simulink model "BLDCmotorControl_FOC_R2017b_fixdt_Ffwd"  (R2017b)
settings: Solver=FixedStepDiscrete  StartTime=0  StopTime=0.5  FixedStep=Ts  MaxStep=1e-6  RelTol=1e-6  AbsTol=1e-6  EnableMultiTasking=on
PreLoadFcn:
  | addpath(genpath('01_Libraries'));
  | addpath(genpath('02_Figures'));
InitFcn:
  | init_model;
values from neighbouring files (symbols this model uses):
  a_elecAngle = 60    [init_model_Ffwd.m]
  b_DCLinkCurrAvail = 0    [init_model_Ffwd.m]
  b_diagEna = 1    [init_model_Ffwd.m]
  b_FfwdEna = 1    [init_model_Ffwd.m]
  b_fieldWeakEna = 0    [init_model_Ffwd.m]
  b_selPhaABCurrMeas = 1    [init_model_Ffwd.m]
  cf_currFilt = 0.02    [init_model_Ffwd.m]
  cf_speedCoef = round(f_ctrl * a_mechAngle * (pi/180) * (30/pi))    [init_model_Ffwd.m]
  cf_speedFilt = 0.20    (= 0.2)    [init_model_Ffwd.m]
  CTRL_COM = 0    [init_model_Ffwd.m]
  dV_openRate = 1000 * Ts_ctrl    (= 0.06)    [init_model_Ffwd.m]
  dz_cntTrnsDetHi = 40    [init_model_Ffwd.m]
  dz_cntTrnsDetLo = 20    [init_model_Ffwd.m]
  i_errThres = 40 * i_sca    (= 2000)    [init_model_Ffwd.m]
  i_max = i_max * i_sca    (= 750)    [init_model_Ffwd.m]
  i_thresOutlier = 200    [init_model_Ffwd.m]
  id_fieldWeak_M1 = [  0   0  0.05  0.25    1    2    3    4  4.5  4.8   5   5] * i_sca    [init_model_Ffwd.m]
  id_Kb = 1000 * Ts_ctrl    (= 0.06)    [init_model_Ffwd.m]
  id_Ki = 80 * Ts_ctrl    (= 0.0048)    [init_model_Ffwd.m]
  id_Kp = 0.5    [init_model_Ffwd.m]
  iq_Kb = 1000 * Ts_ctrl    (= 0.06)    [init_model_Ffwd.m]
  iq_Ki = 100 * Ts_ctrl    (= 0.006)    [init_model_Ffwd.m]
  iq_KiLimProt = 3 * Ts_ctrl    (= 0.00018)    [init_model_Ffwd.m]
  iq_Kp = 0.5    [init_model_Ffwd.m]
  iq_KpLimProt = 4    [init_model_Ffwd.m]
  iq_max_M1 = sqrt(i_max^2 - iq_max_XA.^2)    [init_model_Ffwd.m]
  Ld = 0.00024368    [pe_electric_engine_dyno_data.m]
  Lq = 0.00029758    [pe_electric_engine_dyno_data.m]
  mot_lambda = 0    [init_model_Ffwd.m]
  mot_Ld = 0    [init_model_Ffwd.m]
  mot_Lq = 0    [init_model_Ffwd.m]
  n_commAcvLo = 15    [init_model_Ffwd.m]
  n_commDeacvHi = 30    [init_model_Ffwd.m]
  n_Kb = 1000 * Ts_ctrl    (= 0.06)    [init_model_Ffwd.m]
  n_Ki = 10 * Ts_ctrl    (= 0.0006)    [init_model_Ffwd.m]
  n_Kp = 1    [init_model_Ffwd.m]
  n_KpLimProt = 5    [init_model_Ffwd.m]
  n_max = 800    [init_model_Ffwd.m]
  n_stdStillDet = 3    [init_model_Ffwd.m]
  OPEN_MODE = 0    [init_model_Ffwd.m]
  r_cos_M1 = cos((a_elecAngle_XA + 30)*(pi/180))    [init_model_Ffwd.m]
  r_sin_M1 = sin((a_elecAngle_XA + 30)*(pi/180))    [init_model_Ffwd.m]
  r_whl = 6.5 * 2.54 * 1e-2 / 2    (= 0.08255)    [init_model_Ffwd.m]
  Rs = 0.010087    [pe_electric_engine_dyno_data.m]
  SPD_MODE = 2    [init_model_Ffwd.m]
  t_errDequal = 2 * f_ctrl    (= 32000)    [init_model_Ffwd.m]
  t_errQual = 0.8 * f_ctrl    (= 12800)    [init_model_Ffwd.m]
  TRQ_MODE = 3    [init_model_Ffwd.m]
  Ts = 5e-6    (= 5e-06)    [init_model_Ffwd.m]    (also in pe_electric_engine_dyno_data.m = 1e-05)
  Ts_ctrl = 6e-5    (= 6e-05)    [init_model_Ffwd.m]
  Vd_max = 1000 - V_margin    (= 900)    [init_model_Ffwd.m]
  vec_hallToPos = [0 2 0 1 4 3 5 0]    [init_model_Ffwd.m]
  VLT_MODE = 1    [init_model_Ffwd.m]
  Vq_max_M1 = sqrt(Vd_max^2 - Vq_max_XA.^2)    [init_model_Ffwd.m]
  z_commutMap_M1 = [-1 -1  0  1  1  0 ... (first row only)    [init_model_Ffwd.m]
  z_ctrlModReq = 1    [init_model_Ffwd.m]
  z_ctrlTypSel = 1    [init_model_Ffwd.m]
  z_maxCntRst = 2000    [init_model_Ffwd.m]
undefined symbols (not defined in the file or in its folder): DiscIntNeverNeededParam, sigbuilder_block, V_max, V_min
libraries: powerlib x14, BLDC_controller_Lib x12, simulink x11, pePwmGenerator x1
(part 3 of 3)

== system BLDCmotorControl_FOC_R2017b_fixdt_Ffwd/BLDC_controller/BLDC_controller/F04_Field_Oriented_Control/FeefForward_Decoupling ==
  note: FOC Feedforward Decoupling
      | Vq_Ffwd = n_mot * (mot_Ld*id_Tgt + mot_lambda)
      | Vd_Ffwd = -n_mot * mot_Lq * iq
  n_mot : Inport
  iq_Tgt : Inport  Port=2
  id_Tgt : Inport  Port=3
  Action Port : ActionPort  InitializeStates=reset  ActionType=then
  Divide1 : Product  Inputs=**  RndMeth=Simplest  SaturateOnIntegerOverflow=on  OutDataTypeStr=Inherit: Same as first input
  Divide2 : Product  Inputs=**  OutDataTypeStr=fixdt(1,16,8)  RndMeth=Simplest
  Divide3 : Product  Inputs=**  RndMeth=Simplest  SaturateOnIntegerOverflow=on  OutDataTypeStr=Inherit: Same as first input
  Divide4 : Product  Inputs=**  OutDataTypeStr=fixdt(1,16,8)  RndMeth=Simplest
  Sum6 : Sum  OutDataTypeStr=fixdt(1,16,7)  RndMeth=Simplest
  mot_Ld : Constant  Value=mot_Ld  OutDataTypeStr=fixdt(0,16,16)
  mot_Lq : Constant  Value=mot_Lq  OutDataTypeStr=fixdt(0,16,16)
  mot_lambda : Constant  Value=mot_lambda  OutDataTypeStr=fixdt(0,16,9)
  toNegative : Gain  Tag=struct('comment',struct('text','','placement',1),'logdata',struct('maxnumvals',inf,'plotchannels',[],'loggingmode',3,'channels',1),'output',struct('variable','','description','','name','$S_$B','width',1,'address','','max',NaN,'min',NaN,'class','default','type','CONTINUOUS','scaling','','lsb',1,'offset',0,'arb',0,'freeze',1,'unit','','autoscalingmode',1,'lowerheadroom',1,'upperheadroom',1,'headroomunit','bit','keepdatatype',1,'checkmin',0,'checkmax',0,'castoutput',0,'show',0),'gain',struct('variable','','description','','name','$S_$B_gain','width',1,'address','','max',NaN,'min',NaN,'class','default','type','CONTINUOUS','scaling','','lsb',1,'offset',0,'arb',0,'freeze',1,'unit','','keepdatatype',1,'value','1','scalar',0,'tolerance',1),'scalingvalid',0,'date',730486)  Gain=-1  RndMeth=Zero  OutDataTypeStr=Inherit: Same as input  ParamDataTypeStr=Inherit: Same as input
  Vq_Ffwd : Outport  OutputWhenDisabled=reset  InitialOutput=0
  Vd_Ffwd : Outport  Port=2  OutputWhenDisabled=reset  InitialOutput=0
  wires:
  n_mot/1 -> [n_mot]
  iq_Tgt/1 -> [iq_Tgt]
  id_Tgt/1 -> [id_Tgt]
  Divide1/1 -> toNegative/1
  mot_Ld/1 -> Divide2/2
  [id_Tgt] -> Divide2/1
  Divide2/1 -> Sum6/1
  toNegative/1 -> Vd_Ffwd/1
  mot_lambda/1 -> Sum6/2
  Sum6/1 -> Divide3/2
  [n_mot] -> Divide3/1
  Divide3/1 -> Vq_Ffwd/1
  mot_Lq/1 -> Divide4/2
  [n_mot] -> Divide1/1
  Divide4/1 -> Divide1/2
  [iq_Tgt] -> Divide4/1

== system BLDCmotorControl_FOC_R2017b_fixdt_Ffwd/BLDC_controller/BLDC_controller/F04_Field_Oriented_Control/Field_Weakening ==
  note: Sine/Cosine Look-up Tables
  note: FOC Field weakening
  note: Note: The Sine and Cosine maps are shifted in phase by 30 deg to align with the Hall sensors position.
  note: Field Weakening map as a function of Motor Speed
  a_elecAngle : Inport
  n_motAbs : Inport  Port=2
  Data Type Conversion : DataTypeConversion  OutDataTypeStr=fixdt(1,16,4)
  Switch1 : Switch  Criteria=u2 ~= 0  OutDataTypeStr=Inherit: Inherit via back propagation  RndMeth=Zero
  a_elecAngle_XA : PreLookup  BreakpointsData=a_elecAngle_XA  OutputSelection=Index only  IndexSearchMethod=Evenly spaced points  BeginIndexSearchUsingPreviousIndexResult=on  IndexDataTypeStr=uint8  FractionDataTypeStr=fixdt(0,16,14)  RndMeth=Simplest
  a_elecPeriod1 : Constant  Value=0  OutDataTypeStr=Inherit: Inherit via back propagation
  a_elecPeriod3 : Constant  Value=0  OutDataTypeStr=uint8
  b_fieldWeakEna : Constant  Value=b_fieldWeakEna  OutDataTypeStr=boolean
  id_fieldWeak_M1 : Interpolation_n-D  NumberOfTableDimensions=1  Table=id_fieldWeak_M1  ExtrapMethod=Clip  OutDataTypeStr=fixdt(0,10,0)  InternalRulePriority=Speed  RndMeth=Simplest
      settings: InputPortMap=u0,u1
  n_fieldWeak_XA : PreLookup  BreakpointsData=n_fieldWeak_XA  IndexSearchMethod=Evenly spaced points  BeginIndexSearchUsingPreviousIndexResult=on  IndexDataTypeStr=uint8  FractionDataTypeStr=fixdt(0,8,6)  RndMeth=Simplest
  r_cos_M1 : Interpolation_n-D  NumberOfTableDimensions=1  Table=r_cos_M1  InterpMethod=Flat  ExtrapMethod=Clip  ValidIndexMayReachLast=on  OutDataTypeStr=fixdt(1,16,14)  InternalRulePriority=Speed  RndMeth=Simplest
      settings: InputPortMap=u0,u1
  r_sin_M1 : Interpolation_n-D  NumberOfTableDimensions=1  Table=r_sin_M1  InterpMethod=Flat  ExtrapMethod=Clip  ValidIndexMayReachLast=on  OutDataTypeStr=fixdt(1,16,14)  InternalRulePriority=Speed  RndMeth=Simplest
      settings: InputPortMap=u0,u1
  toNegative : Gain  Tag=struct('comment',struct('text','','placement',1),'logdata',struct('maxnumvals',inf,'plotchannels',[],'loggingmode',3,'channels',1),'output',struct('variable','','description','','name','$S_$B','width',1,'address','','max',NaN,'min',NaN,'class','default','type','CONTINUOUS','scaling','','lsb',1,'offset',0,'arb',0,'freeze',1,'unit','','autoscalingmode',1,'lowerheadroom',1,'upperheadroom',1,'headroomunit','bit','keepdatatype',1,'checkmin',0,'checkmax',0,'castoutput',0,'show',0),'gain',struct('variable','','description','','name','$S_$B_gain','width',1,'address','','max',NaN,'min',NaN,'class','default','type','CONTINUOUS','scaling','','lsb',1,'offset',0,'arb',0,'freeze',1,'unit','','keepdatatype',1,'value','1','scalar',0,'tolerance',1),'scalingvalid',0,'date',730486)  Gain=-1  OutDataTypeStr=fixdt(1,16,4)  RndMeth=Zero  ParamDataTypeStr=Inherit: Same as input
  r_sin : Outport
  r_cos : Outport  Port=2
  id_Tgt : Outport  Port=3
  id_TgtAbs : Outport  Port=4
  wires:
  a_elecAngle_XA/1 -> r_cos_M1/1, r_sin_M1/1
  r_sin_M1/1 -> r_sin/1
  a_elecAngle/1 -> a_elecAngle_XA/1
  r_cos_M1/1 -> r_cos/1
  a_elecPeriod3/1 -> r_cos_M1/2, r_sin_M1/2
  n_fieldWeak_XA/1 -> id_fieldWeak_M1/1
  id_fieldWeak_M1/1 -> Data Type Conversion/1
  n_fieldWeak_XA/2 -> id_fieldWeak_M1/2
  b_fieldWeakEna/1 -> Switch1/2
  Switch1/1 -> id_TgtAbs/1, toNegative/1
  Data Type Conversion/1 -> Switch1/1
  a_elecPeriod1/1 -> Switch1/3
  n_motAbs/1 -> n_fieldWeak_XA/1
  toNegative/1 -> id_Tgt/1

== system BLDCmotorControl_FOC_R2017b_fixdt_Ffwd/BLDC_controller/BLDC_controller/F04_Field_Oriented_Control/Inv_Clarke_Transform ==
  note: Inverse Clarke Transform:
      | V_phaA = V_alpha
      | V_phaB = -(1/2)*V_alpha + (sqrt(3)/2)*V_beta
      | V_phaC = -VphaA - V_phaB
  note: Space Vector Modulation (SVM)
  V_alpha : Inport
  V_beta : Inport  Port=2
  Add : Sum
  Add1 : Sum  Inputs=-+  OutDataTypeStr=Inherit: Same as first input
  Demux : Demux  Outputs=3
  Gain1 : Gain  Tag=struct('comment',struct('text','','placement',1),'logdata',struct('maxnumvals',inf,'plotchannels',[],'loggingmode',3,'channels',1),'output',struct('variable','','description','','name','$S_$B','width',1,'address','','max',NaN,'min',NaN,'class','default','type','CONTINUOUS','scaling','','lsb',1,'offset',0,'arb',0,'freeze',1,'unit','','autoscalingmode',1,'lowerheadroom',1,'upperheadroom',1,'headroomunit','bit','keepdatatype',1,'checkmin',0,'checkmax',0,'castoutput',0,'show',0),'gain',struct('variable','','description','','name','$S_$B_gain','width',1,'address','','max',NaN,'min',NaN,'class','default','type','CONTINUOUS','scaling','','lsb',1,'offset',0,'arb',0,'freeze',1,'unit','','keepdatatype',1,'value','1','scalar',0,'tolerance',1),'scalingvalid',0,'date',730486)  Gain=sqrt(3)/2  OutDataTypeStr=fixdt(1,16,5)  RndMeth=Zero
  Gain2 : Gain  Gain=0.5  OutDataTypeStr=Inherit: Same as input
  Gain3 : Gain  Tag=struct('comment',struct('text','','placement',1),'logdata',struct('maxnumvals',inf,'plotchannels',[],'loggingmode',3,'channels',1),'output',struct('variable','','description','','name','$S_$B','width',1,'address','','max',NaN,'min',NaN,'class','default','type','CONTINUOUS','scaling','','lsb',1,'offset',0,'arb',0,'freeze',1,'unit','','autoscalingmode',1,'lowerheadroom',1,'upperheadroom',1,'headroomunit','bit','keepdatatype',1,'checkmin',0,'checkmax',0,'castoutput',0,'show',0),'gain',struct('variable','','description','','name','$S_$B_gain','width',1,'address','','max',NaN,'min',NaN,'class','default','type','CONTINUOUS','scaling','','lsb',1,'offset',0,'arb',0,'freeze',1,'unit','','keepdatatype',1,'value','1','scalar',0,'tolerance',1),'scalingvalid',0,'date',730486)  Gain=1/2  OutDataTypeStr=fixdt(1,16,5)  RndMeth=Zero
  Gain4 : Gain  Gain=2/sqrt(3)  OutDataTypeStr=fixdt(1,16,0)
  MinMax1 : MinMax  InputSameDT=on
  MinMax2 : MinMax  Function=max  InputSameDT=on
  Mux4 : Mux  Inputs=3
  Sum2 : Sum  Inputs=--  OutDataTypeStr=fixdt(1,16,4)  RndMeth=Simplest
  Sum6 : Sum  Inputs=-+  OutDataTypeStr=fixdt(1,16,4)  RndMeth=Simplest
  V_phaA : Outport
  V_phaB : Outport  Port=2
  V_phaC : Outport  Port=3
  wires:
  Sum6/1 -> Sum2/2, Mux4/2
  Sum2/1 -> Mux4/3
  Gain1/1 -> Sum6/2
  Gain3/1 -> Sum6/1
  V_alpha/1 -> Gain3/1, Sum2/1, Mux4/1  "alpha"
  V_beta/1 -> Gain1/1  "beta"
  Add/1 -> Gain2/1
  Add1/1 -> Gain4/1
  MinMax1/1 -> Add/1
  Demux/3 -> V_phaC/1
  Demux/2 -> V_phaB/1
  Gain2/1 -> Add1/1
  Demux/1 -> V_phaA/1
  MinMax2/1 -> Add/2
  Mux4/1 -> Add1/2, MinMax2/1, MinMax1/1
  Gain4/1 -> Demux/1

== system BLDCmotorControl_FOC_R2017b_fixdt_Ffwd/BLDC_controller/BLDC_controller/F04_Field_Oriented_Control/Inv_Park_Transform ==
  note: Inverse Park Transform:
      | V_alpha = Vd*cos(angle) - Vq*sin(angle)
      | V_beta = Vd*sin(angle) + Vq*cos(angle)
  Vq : Inport
  Vd : Inport  Port=2
  r_sin : Inport  Port=3
  r_cos : Inport  Port=4
  Divide{1..4} (4 alike) : Product  Inputs=**  OutDataTypeStr=fixdt(1,16,5)  RndMeth=Simplest
  Sum1 : Sum  OutDataTypeStr=fixdt(1,16,4)  RndMeth=Simplest
  Sum6 : Sum  Inputs=+-  OutDataTypeStr=fixdt(1,16,4)  RndMeth=Simplest
  V_alpha : Outport
  V_beta : Outport  Port=2
  wires:
  r_sin/1 -> [r_sin]
  Vd/1 -> [Vd]
  Vq/1 -> [Vq]
  r_cos/1 -> [r_cos]
  [r_cos] -> Divide4/2
  [r_sin] -> Divide1/2
  [Vd] -> Divide4/1
  [r_cos] -> Divide3/2
  Divide1/1 -> Sum6/2
  [Vq] -> Divide1/1
  [Vd] -> Divide2/1
  Divide2/1 -> Sum1/1
  Divide3/1 -> Sum1/2
  [Vq] -> Divide3/1
  Divide4/1 -> Sum6/1
  [r_sin] -> Divide2/2
  Sum1/1 -> V_beta/1
  Sum6/1 -> V_alpha/1

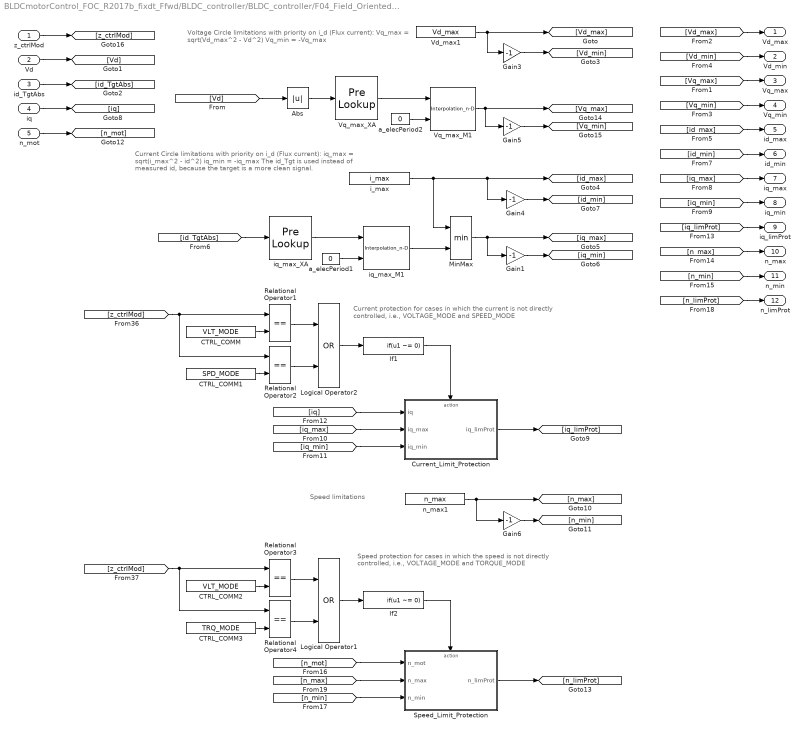
== system BLDCmotorControl_FOC_R2017b_fixdt_Ffwd/BLDC_controller/BLDC_controller/F04_Field_Oriented_Control/Motor_Limitations ==
  note: Voltage Circle limitations with priority on i_d (Flux current):
      | Vq_max = sqrt(Vd_max^2 - Vd^2)
      | Vq_min = -Vq_max
  note: Current Circle limitations with priority on i_d (Flux current):
      | iq_max = sqrt(i_max^2 - id^2)
      | iq_min = -iq_max
      |
      | The id_Tgt is used instead of measured id, because the target is a more clean signal.
  note: Speed limitations
  note: Current protection
      | for cases in which the current is not directly controlled, i.e., VOLTAGE_MODE and SPEED_MODE
  note: Speed protection
      | for cases in which the speed is not directly controlled, i.e., VOLTAGE_MODE and TORQUE_MODE
  z_ctrlMod : Inport
  Vd : Inport  Port=2
  id_TgtAbs : Inport  Port=3
  iq : Inport  Port=4
  n_mot : Inport  Port=5
  Abs : Abs
  CTRL_COMM : Constant  Value=VLT_MODE  OutDataTypeStr=Inherit: Inherit via back propagation
  CTRL_COMM1 : Constant  Value=SPD_MODE  OutDataTypeStr=Inherit: Inherit via back propagation
  CTRL_COMM2 : Constant  Value=VLT_MODE  OutDataTypeStr=Inherit: Inherit via back propagation
  CTRL_COMM3 : Constant  Value=TRQ_MODE  OutDataTypeStr=Inherit: Inherit via back propagation
  Current_Limit_Protection : Subsystem
  Gain{1,3..6} (5 alike) : Gain  Tag=struct('comment',struct('text','','placement',1),'logdata',struct('maxnumvals',inf,'plotchannels',[],'loggingmode',3,'channels',1),'output',struct('variable','','description','','name','$S_$B','width',1,'address','','max',NaN,'min',NaN,'class','default','type','CONTINUOUS','scaling','','lsb',1,'offset',0,'arb',0,'freeze',1,'unit','','autoscalingmode',1,'lowerheadroom',1,'upperheadroom',1,'headroomunit','bit','keepdatatype',1,'checkmin',0,'checkmax',0,'castoutput',0,'show',0),'gain',struct('variable','','description','','name','$S_$B_gain','width',1,'address','','max',NaN,'min',NaN,'class','default','type','CONTINUOUS','scaling','','lsb',1,'offset',0,'arb',0,'freeze',1,'unit','','keepdatatype',1,'value','1','scalar',0,'tolerance',1),'scalingvalid',0,'date',730486)  Gain=-1  RndMeth=Zero  OutDataTypeStr=Inherit: Same as input  ParamDataTypeStr=Inherit: Same as input
  If1 : If  IfExpression=u1 ~= 0  ShowElse=off
  If2 : If  IfExpression=u1 ~= 0  ShowElse=off
  Logical Operator1 : Logic  Operator=OR  AllPortsSameDT=off  OutDataTypeStr=boolean
  Logical Operator2 : Logic  Operator=OR  AllPortsSameDT=off  OutDataTypeStr=boolean
  MinMax : MinMax  Inputs=2
  Relational Operator{1..4} (4 alike) : RelationalOperator  Operator===  OutDataTypeStr=boolean  RndMeth=Simplest
  Speed_Limit_Protection : Subsystem
  Vd_max1 : Constant  Value=Vd_max  OutDataTypeStr=fixdt(1,16,4)
  Vq_max_M1 : Interpolation_n-D  NumberOfTableDimensions=1  Table=Vq_max_M1  InterpMethod=Flat  ExtrapMethod=Clip  ValidIndexMayReachLast=on  OutDataTypeStr=fixdt(1,16,4)  InternalRulePriority=Speed  RndMeth=Simplest
      settings: InputPortMap=u0,u1
  Vq_max_XA : PreLookup  BreakpointsData=Vq_max_XA  OutputSelection=Index only  IndexSearchMethod=Evenly spaced points  BeginIndexSearchUsingPreviousIndexResult=on  IndexDataTypeStr=uint8  FractionDataTypeStr=fixdt(0,8,6)  RndMeth=Simplest
  a_elecPeriod1 : Constant  Value=0  OutDataTypeStr=uint8
  a_elecPeriod2 : Constant  Value=0  OutDataTypeStr=uint8
  i_max : Constant  Value=i_max  OutDataTypeStr=fixdt(1,16,4)
  iq_max_M1 : Interpolation_n-D  NumberOfTableDimensions=1  Table=iq_max_M1  InterpMethod=Flat  ExtrapMethod=Clip  ValidIndexMayReachLast=on  OutDataTypeStr=fixdt(1,16,4)  InternalRulePriority=Speed  RndMeth=Simplest
      settings: InputPortMap=u0,u1
  iq_max_XA : PreLookup  BreakpointsData=iq_max_XA  OutputSelection=Index only  IndexSearchMethod=Evenly spaced points  BeginIndexSearchUsingPreviousIndexResult=on  IndexDataTypeStr=uint8  FractionDataTypeStr=fixdt(0,8,6)  RndMeth=Simplest
  n_max1 : Constant  Value=n_max  OutDataTypeStr=fixdt(1,16,4)
  Vd_max : Outport  OutputWhenDisabled=reset  InitialOutput=V_max
  Vd_min : Outport  Port=2  OutputWhenDisabled=reset  InitialOutput=V_min
  Vq_max : Outport  Port=3  OutputWhenDisabled=reset  InitialOutput=V_max
  Vq_min : Outport  Port=4  OutputWhenDisabled=reset  InitialOutput=V_min
  id_max : Outport  Port=5  OutputWhenDisabled=reset  InitialOutput=V_max
  id_min : Outport  Port=6  OutputWhenDisabled=reset  InitialOutput=V_min
  iq_max : Outport  Port=7  OutputWhenDisabled=reset  InitialOutput=V_max
  iq_min : Outport  Port=8  OutputWhenDisabled=reset  InitialOutput=V_min
  iq_limProt : Outport  Port=9  OutputWhenDisabled=reset  InitialOutput=V_min
  n_max : Outport  Port=10  OutputWhenDisabled=reset  InitialOutput=V_max
  n_min : Outport  Port=11  OutputWhenDisabled=reset  InitialOutput=V_min
  n_limProt : Outport  Port=12  OutputWhenDisabled=reset  InitialOutput=V_min
  wires:
  Vq_max_XA/1 -> Vq_max_M1/1
  [Vq_min] -> Vq_min/1
  [Vq_max] -> Vq_max/1
  Gain5/1 -> [Vq_min]
  Vd_max1/1 -> Gain3/1, [Vd_max]
  Abs/1 -> Vq_max_XA/1
  Vd/1 -> [Vd]
  [Vd] -> Abs/1
  id_TgtAbs/1 -> [id_TgtAbs]
  [Vd_max] -> Vd_max/1
  [Vd_min] -> Vd_min/1
  Gain3/1 -> [Vd_min]
  Gain4/1 -> [id_min]
  i_max/1 -> MinMax/1, Gain4/1, [id_max]
  [id_TgtAbs] -> iq_max_XA/1
  MinMax/1 -> [iq_max], Gain1/1
  Gain1/1 -> [iq_min]
  iq_max_XA/1 -> iq_max_M1/1
  [id_min] -> id_min/1
  [id_max] -> id_max/1
  [iq_max] -> iq_max/1
  [iq_min] -> iq_min/1
  iq/1 -> [iq]
  [iq_limProt] -> iq_limProt/1
  n_max1/1 -> [n_max], Gain6/1
  Gain6/1 -> [n_min]
  [n_min] -> n_min/1
  [n_max] -> n_max/1
  n_mot/1 -> [n_mot]
  [n_limProt] -> n_limProt/1
  z_ctrlMod/1 -> [z_ctrlMod]
  Relational Operator1/1 -> Logical Operator2/1
  [z_ctrlMod] -> Relational Operator2/1, Relational Operator1/1
  Logical Operator2/1 -> If1/1
  Relational Operator2/1 -> Logical Operator2/2
  CTRL_COMM/1 -> Relational Operator1/2
  CTRL_COMM1/1 -> Relational Operator2/2
  CTRL_COMM3/1 -> Relational Operator4/2
  CTRL_COMM2/1 -> Relational Operator3/2
  Relational Operator4/1 -> Logical Operator1/2
  Logical Operator1/1 -> If2/1
  [z_ctrlMod] -> Relational Operator3/1, Relational Operator4/1
  Relational Operator3/1 -> Logical Operator1/1
  [iq_max] -> Current_Limit_Protection/2(iq_max)
  [iq] -> Current_Limit_Protection/1(iq)
  [iq_min] -> Current_Limit_Protection/3(iq_min)
  Current_Limit_Protection/1(iq_limProt) -> [iq_limProt]
  [n_max] -> Speed_Limit_Protection/2(n_max)
  [n_mot] -> Speed_Limit_Protection/1(n_mot)
  [n_min] -> Speed_Limit_Protection/3(n_min)
  Speed_Limit_Protection/1(n_limProt) -> [n_limProt]
  If1/1 -> Current_Limit_Protection/Action
  If2/1 -> Speed_Limit_Protection/Action
  iq_max_M1/1 -> MinMax/2
  a_elecPeriod1/1 -> iq_max_M1/2
  Vq_max_M1/1 -> Gain5/1, [Vq_max]
  a_elecPeriod2/1 -> Vq_max_M1/2

== system BLDCmotorControl_FOC_R2017b_fixdt_Ffwd/BLDC_controller/BLDC_controller/F04_Field_Oriented_Control/Open_Mode ==
  note: This will reduce the control command to 0 with a predefined rate.
  Vq_prev : Inport
  Action Port : ActionPort  InitializeStates=reset  ActionType=default
  Constant23 : Constant  Value=0  OutDataTypeStr=Inherit: Inherit via back propagation
  Data Type Conversion : DataTypeConversion  OutDataTypeStr=fixdt(1,28,16)
  Data Type Conversion1 : DataTypeConversion  OutDataTypeStr=fixdt(1,16,4)
  Gain3 : Gain  Tag=struct('comment',struct('text','','placement',1),'logdata',struct('maxnumvals',inf,'plotchannels',[],'loggingmode',3,'channels',1),'output',struct('variable','','description','','name','$S_$B','width',1,'address','','max',NaN,'min',NaN,'class','default','type','CONTINUOUS','scaling','','lsb',1,'offset',0,'arb',0,'freeze',1,'unit','','autoscalingmode',1,'lowerheadroom',1,'upperheadroom',1,'headroomunit','bit','keepdatatype',1,'checkmin',0,'checkmax',0,'castoutput',0,'show',0),'gain',struct('variable','','description','','name','$S_$B_gain','width',1,'address','','max',NaN,'min',NaN,'class','default','type','CONTINUOUS','scaling','','lsb',1,'offset',0,'arb',0,'freeze',1,'unit','','keepdatatype',1,'value','1','scalar',0,'tolerance',1),'scalingvalid',0,'date',730486)  Gain=-1  RndMeth=Zero  OutDataTypeStr=Inherit: Same as input
  Rate_Limiter : BLDC_controller_Lib/Rate_Limiter  SystemSampleTime=-1
  dV_openRate : Constant  Value=dV_openRate  OutDataTypeStr=fixdt(1,28,16)
  rising_edge_init : BLDC_controller_Lib/rising_edge_init
  Vq_Open : Outport
  wires:
  Vq_prev/1 -> [Vq_prev]
  Constant23/1 -> Rate_Limiter/1
  rising_edge_init/1 -> Rate_Limiter/3
  Gain3/1 -> Rate_Limiter/5
  dV_openRate/1 -> Gain3/1, Rate_Limiter/4
  Data Type Conversion1/1 -> [Vq_Open]
  [Vq_Open] -> Vq_Open/1
  Rate_Limiter/1 -> Data Type Conversion1/1
  [Vq_prev] -> Data Type Conversion/1
  Data Type Conversion/1 -> Rate_Limiter/2

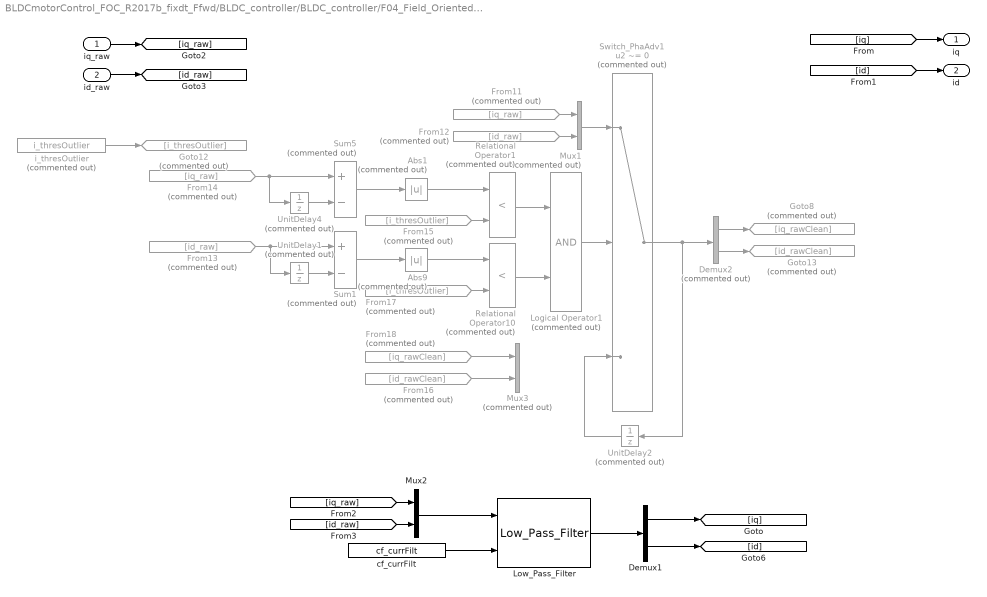
== system BLDCmotorControl_FOC_R2017b_fixdt_Ffwd/BLDC_controller/BLDC_controller/F04_Field_Oriented_Control/Outliers_Removal_and_Filtering ==
  iq_raw : Inport
  id_raw : Inport  Port=2
  Abs1 : Abs  Commented=on
  Abs9 : Abs  Commented=on
  Demux1 : Demux  Outputs=2
  Demux2 : Demux  Commented=on  Outputs=2
  From11 : From  Commented=on  GotoTag=iq_raw
  From12 : From  Commented=on  GotoTag=id_raw
  From13 : From  Commented=on  GotoTag=id_raw
  From14 : From  Commented=on  GotoTag=iq_raw
  From15 : From  Commented=on  GotoTag=i_thresOutlier
  From16 : From  Commented=on  GotoTag=id_rawClean
  From17 : From  Commented=on  GotoTag=i_thresOutlier
  From18 : From  Commented=on  GotoTag=iq_rawClean
  Goto12 : Goto  Commented=on  GotoTag=i_thresOutlier
  Goto13 : Goto  Commented=on  GotoTag=id_rawClean
  Goto8 : Goto  Commented=on  GotoTag=iq_rawClean
  Logical Operator1 : Logic  Commented=on  AllPortsSameDT=off  OutDataTypeStr=boolean
  Low_Pass_Filter : BLDC_controller_Lib/Low_Pass_Filter  SystemSampleTime=-1
  Mux1 : Mux  Commented=on  Inputs=2
  Mux2 : Mux  Inputs=2
  Mux3 : Mux  Commented=on  Inputs=2
  Relational Operator1 : RelationalOperator  Commented=on  Operator=<  OutDataTypeStr=boolean  RndMeth=Simplest
  Relational Operator10 : RelationalOperator  Commented=on  Operator=<  OutDataTypeStr=boolean  RndMeth=Simplest
  Sum1 : Sum  Commented=on  Inputs=+-  RndMeth=Simplest
  Sum5 : Sum  Commented=on  Inputs=+-  RndMeth=Simplest
  Switch_PhaAdv1 : Switch  Commented=on  Criteria=u2 ~= 0  OutDataTypeStr=Inherit: Inherit via back propagation  RndMeth=Zero
  UnitDelay1 : UnitDelay  Commented=on  SampleTime=-1
      settings: AttributesFormatString=Ini=%<X0>
  UnitDelay2 : UnitDelay  Commented=on  SampleTime=-1
      settings: AttributesFormatString=Ini=%<X0>
  UnitDelay4 : UnitDelay  Commented=on  SampleTime=-1
      settings: AttributesFormatString=Ini=%<X0>
  cf_currFilt : Constant  Value=cf_currFilt  OutDataTypeStr=fixdt(0,16,16)
  i_thresOutlier : Constant  Commented=on  Value=i_thresOutlier  OutDataTypeStr=fixdt(0,16,0)
  iq : Outport
  id : Outport  Port=2
  wires:
  Mux2/1 -> Low_Pass_Filter/1
  Sum1/1 -> Abs9/1
  Demux1/2 -> [id]
  cf_currFilt/1 -> Low_Pass_Filter/2
  UnitDelay4/1 -> Sum5/2
  UnitDelay2/1 -> Switch_PhaAdv1/3
  Abs1/1 -> Relational Operator1/1
  From17/1 -> Relational Operator10/2
  Relational Operator1/1 -> Logical Operator1/1
  Abs9/1 -> Relational Operator10/1
  Demux2/1 -> Goto8/1
  Switch_PhaAdv1/1 -> UnitDelay2/1, Demux2/1
  Demux2/2 -> Goto13/1
  From14/1 -> UnitDelay4/1, Sum5/1
  UnitDelay1/1 -> Sum1/2
  i_thresOutlier/1 -> Goto12/1
  From16/1 -> Mux3/2
  Mux1/1 -> Switch_PhaAdv1/1
  From15/1 -> Relational Operator1/2
  From12/1 -> Mux1/2
  From13/1 -> UnitDelay1/1, Sum1/1
  From11/1 -> Mux1/1
  id_raw/1 -> [id_raw]
  Relational Operator10/1 -> Logical Operator1/2
  Logical Operator1/1 -> Switch_PhaAdv1/2
  From18/1 -> Mux3/1
  [iq] -> iq/1
  [id] -> id/1
  iq_raw/1 -> [iq_raw]
  Sum5/1 -> Abs1/1
  Demux1/1 -> [iq]
  Low_Pass_Filter/1 -> Demux1/1
  [iq_raw] -> Mux2/1
  [id_raw] -> Mux2/2

== system BLDCmotorControl_FOC_R2017b_fixdt_Ffwd/BLDC_controller/BLDC_controller/F04_Field_Oriented_Control/Park_Transform ==
  note: Park Transform:
      | iq = -i_alpha*sin(angle) + i_beta*cos(angle)
      | id = i_alpha*cos(angle) + i_beta*sin(angle)
  i_apha : Inport
  i_beta : Inport  Port=2
  r_sin : Inport  Port=3
  r_cos : Inport  Port=4
  Divide{1..4} (4 alike) : Product  Inputs=**  RndMeth=Simplest  OutDataTypeStr=Inherit: Same as first input
  Sum1 : Sum  OutDataTypeStr=fixdt(1,16,4)  RndMeth=Simplest  SaturateOnIntegerOverflow=on
  Sum6 : Sum  Inputs=-+  OutDataTypeStr=fixdt(1,16,4)  RndMeth=Simplest  SaturateOnIntegerOverflow=on
  iq : Outport
  id : Outport  Port=2
  wires:
  r_sin/1 -> [r_sin]
  i_beta/1 -> [i_beta]
  i_apha/1 -> [i_apha]
  r_cos/1 -> [r_cos]
  [r_sin] -> Divide4/2
  [i_apha] -> Divide4/1
  Divide4/1 -> Sum6/1
  Divide1/1 -> Sum6/2
  [i_beta] -> Divide1/1
  [r_cos] -> Divide1/2
  Sum6/1 -> iq/1
  Divide2/1 -> Sum1/1
  [i_apha] -> Divide2/1
  [r_cos] -> Divide2/2
  Divide3/1 -> Sum1/2
  [i_beta] -> Divide3/1
  [r_sin] -> Divide3/2
  Sum1/1 -> id/1

== system BLDCmotorControl_FOC_R2017b_fixdt_Ffwd/BLDC_controller/BLDC_controller/F04_Field_Oriented_Control/Speed_Mode ==
  note: This product is necessary because the value is an input to the Integral part of the PI controller
  r_inpTgtSca : Inport
  Vq_Ffwd : Inport  Port=2
  Vq_max : Inport  Port=3
  Vq_min : Inport  Port=4
  n_mot : Inport  Port=5
  n_max : Inport  Port=6
  n_min : Inport  Port=7
  iq_limProt : Inport  Port=8
  Action Port : ActionPort  InitializeStates=reset  ActionType=case
  Divide1 : Product  Inputs=**  OutDataTypeStr=fixdt(1,16,10)  RndMeth=Simplest
  PI_backCalc_fixdt_n : BLDC_controller_Lib/PI_backCalc_fixdt  SystemSampleTime=-1
  Saturation Dynamic1 : simulink/Discontinuities/Saturation Dynamic  OutMin=[]  OutMax=[]  OutDataTypeStr=Inherit: Same as second input  OutDataType=fixdt(1, 16)  OutScaling=2^-10  DoSatur=off
  Signal Conversion2 : SignalConversion  OverrideOpt=off
  Sum3 : Sum  Inputs=|+-  RndMeth=Simplest
  Terminator : Terminator
      settings: Tag=Controls_Lib  Description=Terminator  CopyFcn=Lib_CopyFcn(gcb);  PreDeleteFcn=Lib_PreDeleteFcn(gcb);
  iq_KiLimProt : Constant  Value=iq_KiLimProt  OutDataTypeStr=fixdt(0,16,16)
  n_Kb : Constant  Value=n_Kb  OutDataTypeStr=fixdt(0,16,16)
  n_Ki : Constant  Value=n_Ki  VectorParams1D=off  OutDataTypeStr=fixdt(0,16,16)
  n_Kp : Constant  Value=n_Kp  OutDataTypeStr=fixdt(0,16,8)
  Vq_Spd : Outport
  wires:
  [Vq_min] -> PI_backCalc_fixdt_n/8
  [Vq_max] -> PI_backCalc_fixdt_n/7
  n_Ki/1 -> PI_backCalc_fixdt_n/4
  n_Kb/1 -> PI_backCalc_fixdt_n/5
  n_Kp/1 -> PI_backCalc_fixdt_n/3
  [n_mot] -> Sum3/2
  Sum3/1 -> PI_backCalc_fixdt_n/2
  r_inpTgtSca/1 -> [r_inpTgtSca]
  Vq_max/1 -> [Vq_max]
  Vq_min/1 -> [Vq_min]
  n_mot/1 -> [n_mot]
  [n_min] -> Saturation Dynamic1/3
  [n_max] -> Saturation Dynamic1/1
  [r_inpTgtSca] -> Saturation Dynamic1/2
  Saturation Dynamic1/1 -> Sum3/1
  n_min/1 -> [n_min]
  n_max/1 -> [n_max]
  PI_backCalc_fixdt_n/1 -> Signal Conversion2/1
  iq_limProt/1 -> [iq_limProt]
  Divide1/1 -> PI_backCalc_fixdt_n/6
  iq_KiLimProt/1 -> Divide1/2
  [iq_limProt] -> Divide1/1
  Signal Conversion2/1 -> Vq_Spd/1
  Vq_Ffwd/1 -> [Vq_Ffwd]
  [Vq_Ffwd] -> PI_backCalc_fixdt_n/1
  PI_backCalc_fixdt_n/2 -> Terminator/1

== system BLDCmotorControl_FOC_R2017b_fixdt_Ffwd/BLDC_controller/BLDC_controller/F04_Field_Oriented_Control/Torque_Mode ==
  r_inpTgtSca : Inport
  Vq_Ffwd : Inport  Port=2
  Vq_max : Inport  Port=3
  Vq_min : Inport  Port=4
  iq : Inport  Port=5
  iq_max : Inport  Port=6
  iq_min : Inport  Port=7
  n_limProt : Inport  Port=8
  Action Port : ActionPort  InitializeStates=reset  ActionType=case
  PI_backCalc_fixdt_Iq : BLDC_controller_Lib/PI_backCalc_fixdt  SystemSampleTime=-1
  Saturation Dynamic : simulink/Discontinuities/Saturation Dynamic  OutMin=[]  OutMax=[]  OutDataTypeStr=Inherit: Same as second input  OutDataType=fixdt(1, 16)  OutScaling=2^-10  DoSatur=off
  Signal Conversion2 : SignalConversion  OverrideOpt=off
  Sum1 : Sum  Inputs=|+-  RndMeth=Simplest
  Sum2 : Sum  RndMeth=Simplest
  constant : Constant  Value=0  OutDataTypeStr=Inherit: Inherit via back propagation
  iq_Kb : Constant  Value=iq_Kb  OutDataTypeStr=fixdt(0,16,16)
  iq_Ki : Constant  Value=iq_Ki  OutDataTypeStr=fixdt(0,16,16)
  iq_Kp : Constant  Value=iq_Kp  OutDataTypeStr=fixdt(0,16,8)
  Vq_Trq : Outport
  Vq_I : Outport  Port=2
  iq_Tgt : Outport  Port=3  OutputWhenDisabled=reset  InitialOutput=0
  wires:
  iq_Ki/1 -> PI_backCalc_fixdt_Iq/4
  [r_inpTgtSca] -> Sum2/1
  [Vq_max] -> PI_backCalc_fixdt_Iq/7
  [Vq_min] -> PI_backCalc_fixdt_Iq/8
  [iq] -> Sum1/2
  Sum1/1 -> PI_backCalc_fixdt_Iq/2
  iq_Kb/1 -> PI_backCalc_fixdt_Iq/5
  iq_Kp/1 -> PI_backCalc_fixdt_Iq/3
  Vq_max/1 -> [Vq_max]
  r_inpTgtSca/1 -> [r_inpTgtSca]
  Vq_min/1 -> [Vq_min]
  iq/1 -> [iq]
  PI_backCalc_fixdt_Iq/1 -> Signal Conversion2/1
  iq_min/1 -> [iq_min]
  iq_max/1 -> [iq_max]
  [iq_min] -> Saturation Dynamic/3
  [iq_max] -> Saturation Dynamic/1
  Sum2/1 -> Saturation Dynamic/2
  [n_limProt] -> Sum2/2
  n_limProt/1 -> [n_limProt]
  constant/1 -> PI_backCalc_fixdt_Iq/6
  Signal Conversion2/1 -> Vq_Trq/1
  Vq_Ffwd/1 -> [Vq_Ffwd]
  [Vq_Ffwd] -> PI_backCalc_fixdt_Iq/1
  PI_backCalc_fixdt_Iq/2 -> Vq_I/1
  Saturation Dynamic/1 -> iq_Tgt/1, Sum1/1

== system BLDCmotorControl_FOC_R2017b_fixdt_Ffwd/BLDC_controller/BLDC_controller/F04_Field_Oriented_Control/Vd_Calculation ==
  id_Tgt : Inport
  id : Inport  Port=2
  Vd_Ffwd : Inport  Port=3
  Vd_max : Inport  Port=4
  Vd_min : Inport  Port=5
  id_max : Inport  Port=6
  id_min : Inport  Port=7
  Action Port : ActionPort  InitializeStates=reset  ActionType=then
  PI_backCalc_fixdt_Id : BLDC_controller_Lib/PI_backCalc_fixdt  SystemSampleTime=-1
  Saturation Dynamic : simulink/Discontinuities/Saturation Dynamic  OutMin=[]  OutMax=[]  OutDataTypeStr=Inherit: Same as second input  OutDataType=fixdt(1, 16)  OutScaling=2^-10  DoSatur=off
  Sum3 : Sum  Inputs=|+-  RndMeth=Simplest
  constant : Constant  Value=0  OutDataTypeStr=Inherit: Inherit via back propagation
  id_Kb : Constant  Value=id_Kb  OutDataTypeStr=fixdt(0,16,16)
  id_Ki : Constant  Value=id_Ki  OutDataTypeStr=fixdt(0,16,16)
  id_Kp : Constant  Value=id_Kp  OutDataTypeStr=fixdt(0,16,8)
  Vd : Outport  OutputWhenDisabled=reset  InitialOutput=0
  Vd_I : Outport  Port=2  OutputWhenDisabled=reset  InitialOutput=0
  wires:
  [id] -> Sum3/2
  [id_Tgt] -> Saturation Dynamic/2
  id_Tgt/1 -> [id_Tgt]
  id/1 -> [id]
  Vd_min/1 -> [Vd_min]
  Vd_max/1 -> [Vd_max]
  id_max/1 -> [id_max]
  id_min/1 -> [id_min]
  Saturation Dynamic/1 -> Sum3/1
  [id_max] -> Saturation Dynamic/1
  [id_min] -> Saturation Dynamic/3
  Sum3/1 -> PI_backCalc_fixdt_Id/2
  Vd_Ffwd/1 -> [Vd_Ffwd]
  [Vd_Ffwd] -> PI_backCalc_fixdt_Id/1
  [Vd_max] -> PI_backCalc_fixdt_Id/7
  [Vd_min] -> PI_backCalc_fixdt_Id/8
  id_Kp/1 -> PI_backCalc_fixdt_Id/3
  id_Ki/1 -> PI_backCalc_fixdt_Id/4
  id_Kb/1 -> PI_backCalc_fixdt_Id/5
  constant/1 -> PI_backCalc_fixdt_Id/6
  PI_backCalc_fixdt_Id/1 -> Vd/1
  PI_backCalc_fixdt_Id/2 -> Vd_I/1

== system BLDCmotorControl_FOC_R2017b_fixdt_Ffwd/BLDC_controller/BLDC_controller/F04_Field_Oriented_Control/Voltage_Mode ==
  r_inpTgtSca : Inport
  Vq_Ffwd : Inport  Port=2
  Vq_max : Inport  Port=3
  Vq_min : Inport  Port=4
  iq_limProt : Inport  Port=5
  n_limProt : Inport  Port=6
  Action Port : ActionPort  InitializeStates=reset  ActionType=case
  Saturation Dynamic1 : simulink/Discontinuities/Saturation Dynamic  OutMin=[]  OutMax=[]  OutDataTypeStr=Inherit: Same as second input  OutDataType=fixdt(1, 16)  OutScaling=2^-10  DoSatur=off
  Signal Conversion2 : SignalConversion  OverrideOpt=off
  Sum3 : Sum  Inputs=++++  RndMeth=Simplest
  Vq_Vlt : Outport
  wires:
  r_inpTgtSca/1 -> [r_inpTgtSca]
  [Vq_min] -> Saturation Dynamic1/3
  [Vq_max] -> Saturation Dynamic1/1
  Vq_max/1 -> [Vq_max]
  Vq_min/1 -> [Vq_min]
  iq_limProt/1 -> [iq_limProt]
  n_limProt/1 -> [n_limProt]
  Sum3/1 -> Saturation Dynamic1/2
  Saturation Dynamic1/1 -> Signal Conversion2/1
  [r_inpTgtSca] -> Sum3/1
  Signal Conversion2/1 -> Vq_Vlt/1
  Vq_Ffwd/1 -> [Vq_Ffwd]
  [Vq_Ffwd] -> Sum3/2
  [iq_limProt] -> Sum3/3
  [n_limProt] -> Sum3/4

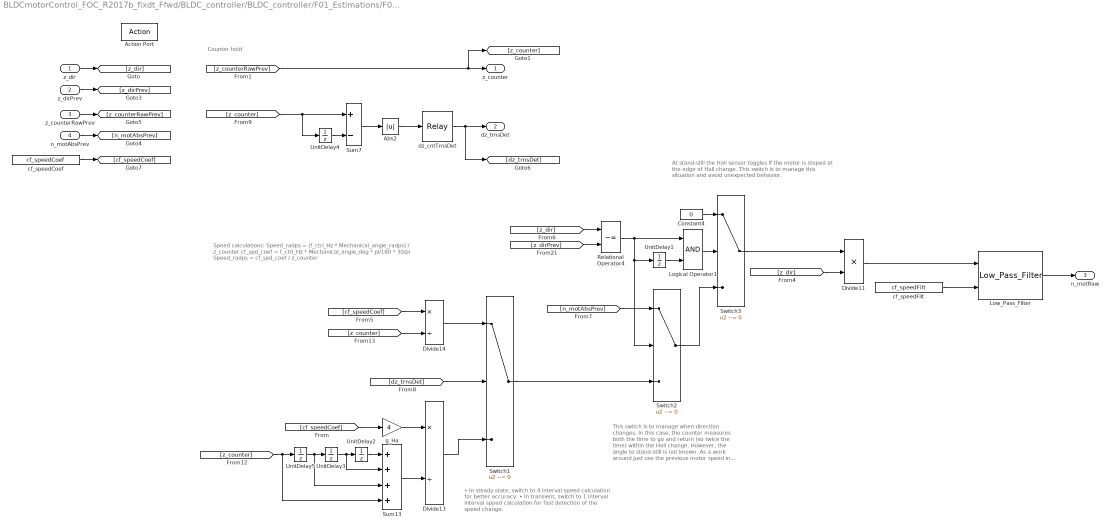
== system BLDCmotorControl_FOC_R2017b_fixdt_Ffwd/BLDC_controller/BLDC_controller/F01_Estimations/F01_04_Speed_Estimation/Raw_Motor_Speed_Estimation ==
  note: Speed calculations:
      | Speed_radps = (f_ctrl_Hz * Mechanical_angle_radps) / z_counter
      | cf_spd_coef = f_ctrl_Hz * Mechanical_angle_deg * pi/180 * 30/pi
      | Speed_radps = cf_spd_coef / z_counter
  note: Counter hold
  note: • In steady state, switch to 4 interval speed calculation for better accuracy.
      | • In transient, switch to 1 interval interval spped calculation for fast detection of the speed change.
  note: This switch is to manage when direction changes. In this case, the counter measures both the time to go and return (so twice the time) within the Hall change. However, the angle to stand-still is not known. As a work around just use the previous motor speed in absolute value.
  note: At stand-still the Hall sensor toggles if the motor is stoped at the edge of Hall change. This switch is to manage this situation and avoid unexpected behavior.
  z_dir : Inport
  z_dirPrev : Inport  Port=2
  z_counterRawPrev : Inport  Port=3
  n_motAbsPrev : Inport  Port=4
  Action Port : ActionPort  ActionType=then
  Abs2 : Abs  OutDataTypeStr=Inherit: Inherit via back propagation  RndMeth=Zero
  Constant4 : Constant  Value=0  OutDataTypeStr=Inherit: Inherit via back propagation
  Divide11 : Product  Inputs=**  RndMeth=Simplest  OutDataTypeStr=Inherit: Same as first input
  Divide13 : Product  Inputs=*/  OutDataTypeStr=fixdt(1,16,4)  RndMeth=Simplest
  Divide14 : Product  Inputs=*/  OutDataTypeStr=fixdt(1,16,4)  RndMeth=Simplest
  Logical Operator1 : Logic  AllPortsSameDT=off  OutDataTypeStr=boolean
  Low_Pass_Filter : BLDC_controller_Lib/Low_Pass_Filter  SystemSampleTime=-1
  Relational Operator4 : RelationalOperator  Operator=~=  OutDataTypeStr=boolean  RndMeth=Simplest
  Sum13 : Sum  Inputs=++++  RndMeth=Simplest  InputSameDT=on  OutDataTypeStr=Inherit: Same as first input
  Sum7 : Sum  Inputs=+-  RndMeth=Simplest  InputSameDT=on  OutDataTypeStr=Inherit: Same as first input
  Switch1 : Switch  Tag=struct('comment',struct('text','','placement',1),'logdata',struct('maxnumvals',inf,'plotchannels',[],'loggingmode',3,'channels',1),'output',struct('variable','','description','','name','$S_$B','width',1,'address','','max',NaN,'min',NaN,'class','default','type','CONTINUOUS','scaling','','lsb',1,'offset',0,'arb',0,'freeze',1,'unit','','autoscalingmode',1,'lowerheadroom',1,'upperheadroom',1,'headroomunit','bit','keepdatatype',1,'checkmin',0,'checkmax',0,'castoutput',0,'show',0),'threshold',struct('variable','','description','','name','$S_$B_threshold','width',1,'address','','max',NaN,'min',NaN,'class','default','type','CONTINUOUS','scaling','','lsb',1,'offset',0,'arb',0,'freeze',1,'unit','','keepdatatype',1,'value','0','scalar',0,'criteria',3),'scalingvalid',0,'date',733087.49614628474,'inheritscaling',0)  Criteria=u2 ~= 0  SaturateOnIntegerOverflow=on  InputSameDT=on
      settings: AttributesFormatString=threshold=%<threshold>\nCriteria : %<Criteria>
  Switch2 : Switch  Tag=struct('comment',struct('text','','placement',1),'logdata',struct('maxnumvals',inf,'plotchannels',[],'loggingmode',3,'channels',1),'output',struct('variable','','description','','name','$S_$B','width',1,'address','','max',NaN,'min',NaN,'class','default','type','CONTINUOUS','scaling','','lsb',1,'offset',0,'arb',0,'freeze',1,'unit','','autoscalingmode',1,'lowerheadroom',1,'upperheadroom',1,'headroomunit','bit','keepdatatype',1,'checkmin',0,'checkmax',0,'castoutput',0,'show',0),'threshold',struct('variable','','description','','name','$S_$B_threshold','width',1,'address','','max',NaN,'min',NaN,'class','default','type','CONTINUOUS','scaling','','lsb',1,'offset',0,'arb',0,'freeze',1,'unit','','keepdatatype',1,'value','0','scalar',0,'criteria',3),'scalingvalid',0,'date',733087.49614628474,'inheritscaling',0)  Criteria=u2 ~= 0  SaturateOnIntegerOverflow=on  InputSameDT=on
      settings: AttributesFormatString=threshold=%<threshold>\nCriteria : %<Criteria>
  Switch3 : Switch  Tag=struct('comment',struct('text','','placement',1),'logdata',struct('maxnumvals',inf,'plotchannels',[],'loggingmode',3,'channels',1),'output',struct('variable','','description','','name','$S_$B','width',1,'address','','max',NaN,'min',NaN,'class','default','type','CONTINUOUS','scaling','','lsb',1,'offset',0,'arb',0,'freeze',1,'unit','','autoscalingmode',1,'lowerheadroom',1,'upperheadroom',1,'headroomunit','bit','keepdatatype',1,'checkmin',0,'checkmax',0,'castoutput',0,'show',0),'threshold',struct('variable','','description','','name','$S_$B_threshold','width',1,'address','','max',NaN,'min',NaN,'class','default','type','CONTINUOUS','scaling','','lsb',1,'offset',0,'arb',0,'freeze',1,'unit','','keepdatatype',1,'value','0','scalar',0,'criteria',3),'scalingvalid',0,'date',733087.49614628474,'inheritscaling',0)  Criteria=u2 ~= 0  SaturateOnIntegerOverflow=on  InputSameDT=on
      settings: AttributesFormatString=threshold=%<threshold>\nCriteria : %<Criteria>
  UnitDelay{1..5} (5 alike) : UnitDelay  SampleTime=-1
      settings: AttributesFormatString=Ini=%<X0>
  cf_speedCoef : Constant  Value=cf_speedCoef  OutDataTypeStr=fixdt(0,16,0)
  cf_speedFilt : Constant  Value=cf_speedFilt  OutDataTypeStr=fixdt(0,16,16)
  dz_cntTrnsDet : Relay  OnSwitchValue=dz_cntTrnsDetHi  OffSwitchValue=dz_cntTrnsDetLo  OutDataTypeStr=boolean
  g_Ha : Gain  Gain=4  OutDataTypeStr=Inherit: Inherit via back propagation  RndMeth=Zero  ParamDataTypeStr=Inherit: Same as input
  z_counter : Outport  InitialOutput=z_maxCntRst
  dz_trnsDet : Outport  Port=2
  n_motRaw : Outport  Port=3
  wires:
  z_dir/1 -> [z_dir]
  z_dirPrev/1 -> [z_dirPrev]
  z_counterRawPrev/1 -> [z_counterRawPrev]
  Divide11/1 -> Low_Pass_Filter/1
  [z_dir] -> Divide11/2
  UnitDelay3/1 -> UnitDelay2/1, Sum13/2
  UnitDelay5/1 -> UnitDelay3/1, Sum13/3
  [z_counter] -> UnitDelay5/1, Sum13/4
  [cf_speedCoef] -> g_Ha/1
  Sum13/1 -> Divide13/2
  g_Ha/1 -> Divide13/1
  [z_counter] -> Divide14/2
  [cf_speedCoef] -> Divide14/1
  UnitDelay4/1 -> Sum7/2
  [z_counter] -> UnitDelay4/1, Sum7/1
  Sum7/1 -> Abs2/1
  Abs2/1 -> dz_cntTrnsDet/1
  [dz_trnsDet] -> Switch1/2
  cf_speedCoef/1 -> [cf_speedCoef]
  UnitDelay2/1 -> Sum13/1
  [z_dir] -> Relational Operator4/1
  [z_dirPrev] -> Relational Operator4/2
  UnitDelay1/1 -> Logical Operator1/2
  Relational Operator4/1 -> UnitDelay1/1, Switch2/2, Logical Operator1/1
  Logical Operator1/1 -> Switch3/2
  Switch2/1 -> Switch3/3
  Constant4/1 -> Switch3/1
  Switch3/1 -> Divide11/1
  n_motAbsPrev/1 -> [n_motAbsPrev]
  [n_motAbsPrev] -> Switch2/1
  [z_counterRawPrev] -> [z_counter], z_counter/1
  dz_cntTrnsDet/1 -> [dz_trnsDet], dz_trnsDet/1
  Divide13/1 -> Switch1/3
  cf_speedFilt/1 -> Low_Pass_Filter/2
  Low_Pass_Filter/1 -> n_motRaw/1
  Divide14/1 -> Switch1/1
  Switch1/1 -> Switch2/3

== system BLDCmotorControl_FOC_R2017b_fixdt_Ffwd/BLDC_controller/BLDC_controller/F04_Field_Oriented_Control/Clarke_Transform/Clarke_PhasesAB ==
  note: Clarke Transform:
      | i_alpha = i_phaA
      | i_beta = ((1/sqrt(3))*i_phaA + (2/sqrt(3))*i_phaB)
  i_phaA : Inport
  i_phaB : Inport  Port=2
  Action Port : ActionPort  ActionType=then
  Gain2 : Gain  Tag=struct('comment',struct('text','','placement',1),'logdata',struct('maxnumvals',inf,'plotchannels',[],'loggingmode',3,'channels',1),'output',struct('variable','','description','','name','$S_$B','width',1,'address','','max',NaN,'min',NaN,'class','default','type','CONTINUOUS','scaling','','lsb',1,'offset',0,'arb',0,'freeze',1,'unit','','autoscalingmode',1,'lowerheadroom',1,'upperheadroom',1,'headroomunit','bit','keepdatatype',1,'checkmin',0,'checkmax',0,'castoutput',0,'show',0),'gain',struct('variable','','description','','name','$S_$B_gain','width',1,'address','','max',NaN,'min',NaN,'class','default','type','CONTINUOUS','scaling','','lsb',1,'offset',0,'arb',0,'freeze',1,'unit','','keepdatatype',1,'value','1','scalar',0,'tolerance',1),'scalingvalid',0,'date',730486)  Gain=2/sqrt(3)  RndMeth=Zero  OutDataTypeStr=Inherit: Same as input
  Gain4 : Gain  Tag=struct('comment',struct('text','','placement',1),'logdata',struct('maxnumvals',inf,'plotchannels',[],'loggingmode',3,'channels',1),'output',struct('variable','','description','','name','$S_$B','width',1,'address','','max',NaN,'min',NaN,'class','default','type','CONTINUOUS','scaling','','lsb',1,'offset',0,'arb',0,'freeze',1,'unit','','autoscalingmode',1,'lowerheadroom',1,'upperheadroom',1,'headroomunit','bit','keepdatatype',1,'checkmin',0,'checkmax',0,'castoutput',0,'show',0),'gain',struct('variable','','description','','name','$S_$B_gain','width',1,'address','','max',NaN,'min',NaN,'class','default','type','CONTINUOUS','scaling','','lsb',1,'offset',0,'arb',0,'freeze',1,'unit','','keepdatatype',1,'value','1','scalar',0,'tolerance',1),'scalingvalid',0,'date',730486)  Gain=1/sqrt(3)  RndMeth=Zero  OutDataTypeStr=Inherit: Same as input
  Signal Conversion2 : SignalConversion  OverrideOpt=off
  Sum1 : Sum  OutDataTypeStr=fixdt(1,16,4)  RndMeth=Simplest  SaturateOnIntegerOverflow=on
  i_alphaAB : Outport
  i_betaAB : Outport  Port=2
  wires:
  i_phaB/1 -> [i_phaB]
  i_phaA/1 -> [i_phaA]
  [i_phaA] -> Signal Conversion2/1, Gain4/1
  Gain2/1 -> Sum1/2
  [i_phaB] -> Gain2/1
  Gain4/1 -> Sum1/1
  Sum1/1 -> i_betaAB/1
  Signal Conversion2/1 -> i_alphaAB/1

== system BLDCmotorControl_FOC_R2017b_fixdt_Ffwd/BLDC_controller/BLDC_controller/F04_Field_Oriented_Control/Clarke_Transform/Clarke_PhasesBC ==
  note: Clarke Transform:
      | i_alpha = - i_phaB - i_phaC
      | i_beta = (1/sqrt(3)) * (i_phaB - i_phaC)
  i_phaB : Inport
  i_phaC : Inport  Port=2
  Action Port : ActionPort  ActionType=else
  Gain2 : Gain  Tag=struct('comment',struct('text','','placement',1),'logdata',struct('maxnumvals',inf,'plotchannels',[],'loggingmode',3,'channels',1),'output',struct('variable','','description','','name','$S_$B','width',1,'address','','max',NaN,'min',NaN,'class','default','type','CONTINUOUS','scaling','','lsb',1,'offset',0,'arb',0,'freeze',1,'unit','','autoscalingmode',1,'lowerheadroom',1,'upperheadroom',1,'headroomunit','bit','keepdatatype',1,'checkmin',0,'checkmax',0,'castoutput',0,'show',0),'gain',struct('variable','','description','','name','$S_$B_gain','width',1,'address','','max',NaN,'min',NaN,'class','default','type','CONTINUOUS','scaling','','lsb',1,'offset',0,'arb',0,'freeze',1,'unit','','keepdatatype',1,'value','1','scalar',0,'tolerance',1),'scalingvalid',0,'date',730486)  Gain=1/sqrt(3)  RndMeth=Zero  OutDataTypeStr=Inherit: Same as input
  Sum1 : Sum  Inputs=--  OutDataTypeStr=fixdt(1,16,4)  RndMeth=Simplest  SaturateOnIntegerOverflow=on
  Sum3 : Sum  Inputs=+-  OutDataTypeStr=fixdt(1,16,4)  RndMeth=Simplest  SaturateOnIntegerOverflow=on
  i_alphaBC : Outport
  i_betaBC : Outport  Port=2
  wires:
  [i_phaC] -> Sum1/2
  [i_phaB] -> Sum1/1
  [i_phaC] -> Sum3/2
  Gain2/1 -> i_betaBC/1
  Sum3/1 -> Gain2/1
  [i_phaB] -> Sum3/1
  Sum1/1 -> i_alphaBC/1
  i_phaB/1 -> [i_phaB]
  i_phaC/1 -> [i_phaC]

== system BLDCmotorControl_FOC_R2017b_fixdt_Ffwd/BLDC_controller/BLDC_controller/F04_Field_Oriented_Control/Motor_Limitations/Current_Limit_Protection ==
  iq : Inport
  iq_max : Inport  Port=2
  iq_min : Inport  Port=3
  Action Port : ActionPort  InitializeStates=reset  ActionType=then
  Divide4 : Product  Inputs=**  RndMeth=Simplest  SaturateOnIntegerOverflow=on  OutDataTypeStr=Inherit: Same as first input
  Kp_iqLimProt : Constant  Value=iq_KpLimProt  OutDataTypeStr=fixdt(0,16,6)
  Saturation Dynamic : simulink/Discontinuities/Saturation Dynamic  OutMin=[]  OutMax=[]  OutDataTypeStr=Inherit: Same as second input  OutDataType=fixdt(1, 16)  OutScaling=2^-10  DoSatur=off
  Sum3 : Sum  Inputs=|+-  RndMeth=Simplest
  iq_limProt : Outport  OutputWhenDisabled=reset  InitialOutput=0
  wires:
  Sum3/1 -> Divide4/1
  iq/1 -> Sum3/2, Saturation Dynamic/2
  Kp_iqLimProt/1 -> Divide4/2
  Saturation Dynamic/1 -> Sum3/1
  iq_max/1 -> Saturation Dynamic/1
  iq_min/1 -> Saturation Dynamic/3
  Divide4/1 -> iq_limProt/1

== system BLDCmotorControl_FOC_R2017b_fixdt_Ffwd/BLDC_controller/BLDC_controller/F04_Field_Oriented_Control/Motor_Limitations/Speed_Limit_Protection ==
  n_mot : Inport
  n_max : Inport  Port=2
  n_min : Inport  Port=3
  Action Port : ActionPort  InitializeStates=reset  ActionType=then
  Divide1 : Product  Inputs=**  RndMeth=Simplest  SaturateOnIntegerOverflow=on  OutDataTypeStr=Inherit: Same as first input
  Kp_nLimProt : Constant  Value=n_KpLimProt  OutDataTypeStr=fixdt(0,16,6)
  Saturation Dynamic1 : simulink/Discontinuities/Saturation Dynamic  OutMin=[]  OutMax=[]  OutDataTypeStr=Inherit: Same as second input  OutDataType=fixdt(1, 16)  OutScaling=2^-10  DoSatur=off
  Sum1 : Sum  Inputs=|+-  RndMeth=Simplest
  n_limProt : Outport  OutputWhenDisabled=reset  InitialOutput=0
  wires:
  Saturation Dynamic1/1 -> Sum1/1
  n_min/1 -> Saturation Dynamic1/3
  Sum1/1 -> Divide1/1
  n_max/1 -> Saturation Dynamic1/1
  Kp_nLimProt/1 -> Divide1/2
  n_mot/1 -> Sum1/2, Saturation Dynamic1/2
  Divide1/1 -> n_limProt/1

== stateflow chart BLDCmotorControl_FOC_R2017b_fixdt_Ffwd/BLDC_controller/BLDC_controller/F03_Control_Mode_Manager/F02_02_Control_Mode_Manager ==
  state OPEN
    entry:
    z_ctrlMod = OPEN_MODE;
  state ACTIVE
    state TORQUE_MODE
      entry:
      z_ctrlMod = TRQ_MODE;
    state SPEED_MODE
      entry:
      z_ctrlMod = SPD_MODE;
    state VOLTAGE_MODE
      entry:
      z_ctrlMod = VLT_MODE;
    (default) -> (junction 7)
    (junction 7) -> TORQUE_MODE [order 1] : [b_toTrqMod]
    (junction 7) -> (junction 8) [order 2]
    (junction 8) -> SPEED_MODE [order 1] : [b_toSpdMod]
    (junction 8) -> (junction 29) [order 2]
    (junction 29) -> VOLTAGE_MODE
  (default) -> OPEN
  OPEN -> ACTIVE : [b_toActive]
  ACTIVE -> OPEN : [b_toOpen]
  data: b_toOpen input boolean; b_toActive input boolean; b_toSpdMod input boolean; z_ctrlMod output uint8; OPEN_MODE constant uint8 =OPEN_MODE; TRQ_MODE constant uint8 =TRQ_MODE; SPD_MODE constant uint8 =SPD_MODE; VLT_MODE constant uint8 =VLT_MODE; b_toTrqMod input boolean
